simulink model "BTP_HEV_UDC_fInal_25_11_19"  (R2019a)
settings: Solver=VariableStepAuto  StartTime=0.0  StopTime=100  RelTol=1e-3
undefined symbols (not defined in the file): f_co, f_co2, f_hc, f_nox, f_tbrake_n_bpt, f_tbrake_t_bpt
libraries: fl_lib x100, nesl_utility x32, ee_lib x26, sdl_lib x17, simulink x5
(part 2 of 2)

== system BTP_HEV_UDC_fInal_25_11_19/Motor/Battery Subsystem/Battery Pack Subsystem/battery unit1 ==
  Capacitor : fl_lib/Electrical/Electrical Elements/Capacitor  c=5000 F  r=1e-6 Ohm  g=0 1/Ohm  i_specify=off  i_priority=None  i=0 A  i_nominal_specify=off  i_nominal_unit=A  i_nominal_value=1  v_specify=off  v_priority=None  v=0 V  v_nominal_specify=off  v_nominal_unit=V  v_nominal_value=1  vc_specify=off  vc_priority=High  vc=0 V  vc_nominal_specify=off  vc_nominal_unit=V  vc_nominal_value=1
  DC Voltage Source : ee_lib/Additional Components/SPICE Sources/DC Voltage Source  DC=4 V
      settings: SourceProductName=Simscape Electrical
  Resistor : fl_lib/Electrical/Electrical Elements/Resistor  R=.01 Ohm  i_specify=off  i_priority=None  i=0 A  i_nominal_specify=off  i_nominal_unit=A  i_nominal_value=1  v_specify=off  v_priority=None  v=0 V  v_nominal_specify=off  v_nominal_unit=V  v_nominal_value=1
  Resistor1 : fl_lib/Electrical/Electrical Elements/Resistor  R=.005 Ohm  i_specify=off  i_priority=None  i=0 A  i_nominal_specify=off  i_nominal_unit=A  i_nominal_value=1  v_specify=off  v_priority=None  v=0 V  v_nominal_specify=off  v_nominal_unit=V  v_nominal_value=1
  + : PMIOPort  Side=Right
  - : PMIOPort  Port=2  Side=Left
  connections:
  Resistor/LConn1 -- DC Voltage Source/LConn1
  -/RConn1 -- DC Voltage Source/RConn1
  +/RConn1 -- Capacitor/RConn1 -- Resistor1/RConn1
  Resistor1/LConn1 -- Capacitor/LConn1 -- Resistor/RConn1

== system BTP_HEV_UDC_fInal_25_11_19/Motor/Battery Subsystem/Battery Pack Subsystem/battery unit10 ==
  Capacitor : fl_lib/Electrical/Electrical Elements/Capacitor  c=5000 F  r=1e-6 Ohm  g=0 1/Ohm  i_specify=off  i_priority=None  i=0 A  i_nominal_specify=off  i_nominal_unit=A  i_nominal_value=1  v_specify=off  v_priority=None  v=0 V  v_nominal_specify=off  v_nominal_unit=V  v_nominal_value=1  vc_specify=off  vc_priority=High  vc=0 V  vc_nominal_specify=off  vc_nominal_unit=V  vc_nominal_value=1
  DC Voltage Source : ee_lib/Additional Components/SPICE Sources/DC Voltage Source  DC=4 V
      settings: SourceProductName=Simscape Electrical
  Resistor : fl_lib/Electrical/Electrical Elements/Resistor  R=.01 Ohm  i_specify=off  i_priority=None  i=0 A  i_nominal_specify=off  i_nominal_unit=A  i_nominal_value=1  v_specify=off  v_priority=None  v=0 V  v_nominal_specify=off  v_nominal_unit=V  v_nominal_value=1
  Resistor1 : fl_lib/Electrical/Electrical Elements/Resistor  R=.005 Ohm  i_specify=off  i_priority=None  i=0 A  i_nominal_specify=off  i_nominal_unit=A  i_nominal_value=1  v_specify=off  v_priority=None  v=0 V  v_nominal_specify=off  v_nominal_unit=V  v_nominal_value=1
  + : PMIOPort  Side=Right
  - : PMIOPort  Port=2  Side=Left
  connections:
  Resistor/RConn1 -- Capacitor/LConn1 -- Resistor1/LConn1
  Resistor1/RConn1 -- Capacitor/RConn1 -- +/RConn1
  -/RConn1 -- DC Voltage Source/RConn1
  Resistor/LConn1 -- DC Voltage Source/LConn1

== system BTP_HEV_UDC_fInal_25_11_19/Motor/Battery Subsystem/Battery Pack Subsystem/battery unit11 ==
  Capacitor : fl_lib/Electrical/Electrical Elements/Capacitor  c=5000 F  r=1e-6 Ohm  g=0 1/Ohm  i_specify=off  i_priority=None  i=0 A  i_nominal_specify=off  i_nominal_unit=A  i_nominal_value=1  v_specify=off  v_priority=None  v=0 V  v_nominal_specify=off  v_nominal_unit=V  v_nominal_value=1  vc_specify=off  vc_priority=High  vc=0 V  vc_nominal_specify=off  vc_nominal_unit=V  vc_nominal_value=1
  DC Voltage Source : ee_lib/Additional Components/SPICE Sources/DC Voltage Source  DC=4 V
      settings: SourceProductName=Simscape Electrical
  Resistor : fl_lib/Electrical/Electrical Elements/Resistor  R=.01 Ohm  i_specify=off  i_priority=None  i=0 A  i_nominal_specify=off  i_nominal_unit=A  i_nominal_value=1  v_specify=off  v_priority=None  v=0 V  v_nominal_specify=off  v_nominal_unit=V  v_nominal_value=1
  Resistor1 : fl_lib/Electrical/Electrical Elements/Resistor  R=.005 Ohm  i_specify=off  i_priority=None  i=0 A  i_nominal_specify=off  i_nominal_unit=A  i_nominal_value=1  v_specify=off  v_priority=None  v=0 V  v_nominal_specify=off  v_nominal_unit=V  v_nominal_value=1
  + : PMIOPort  Side=Right
  - : PMIOPort  Port=2  Side=Left
  connections:
  Resistor/LConn1 -- DC Voltage Source/LConn1
  -/RConn1 -- DC Voltage Source/RConn1
  +/RConn1 -- Capacitor/RConn1 -- Resistor1/RConn1
  Resistor1/LConn1 -- Capacitor/LConn1 -- Resistor/RConn1

== system BTP_HEV_UDC_fInal_25_11_19/Motor/Battery Subsystem/Battery Pack Subsystem/battery unit12 ==
  Capacitor : fl_lib/Electrical/Electrical Elements/Capacitor  c=5000 F  r=1e-6 Ohm  g=0 1/Ohm  i_specify=off  i_priority=None  i=0 A  i_nominal_specify=off  i_nominal_unit=A  i_nominal_value=1  v_specify=off  v_priority=None  v=0 V  v_nominal_specify=off  v_nominal_unit=V  v_nominal_value=1  vc_specify=off  vc_priority=High  vc=0 V  vc_nominal_specify=off  vc_nominal_unit=V  vc_nominal_value=1
  DC Voltage Source : ee_lib/Additional Components/SPICE Sources/DC Voltage Source  DC=4 V
      settings: SourceProductName=Simscape Electrical
  Resistor : fl_lib/Electrical/Electrical Elements/Resistor  R=.01 Ohm  i_specify=off  i_priority=None  i=0 A  i_nominal_specify=off  i_nominal_unit=A  i_nominal_value=1  v_specify=off  v_priority=None  v=0 V  v_nominal_specify=off  v_nominal_unit=V  v_nominal_value=1
  Resistor1 : fl_lib/Electrical/Electrical Elements/Resistor  R=.005 Ohm  i_specify=off  i_priority=None  i=0 A  i_nominal_specify=off  i_nominal_unit=A  i_nominal_value=1  v_specify=off  v_priority=None  v=0 V  v_nominal_specify=off  v_nominal_unit=V  v_nominal_value=1
  + : PMIOPort  Side=Right
  - : PMIOPort  Port=2  Side=Left
  connections:
  Resistor/RConn1 -- Capacitor/LConn1 -- Resistor1/LConn1
  Resistor1/RConn1 -- Capacitor/RConn1 -- +/RConn1
  -/RConn1 -- DC Voltage Source/RConn1
  Resistor/LConn1 -- DC Voltage Source/LConn1

== system BTP_HEV_UDC_fInal_25_11_19/Motor/Battery Subsystem/Battery Pack Subsystem/battery unit13 ==
  Capacitor : fl_lib/Electrical/Electrical Elements/Capacitor  c=5000 F  r=1e-6 Ohm  g=0 1/Ohm  i_specify=off  i_priority=None  i=0 A  i_nominal_specify=off  i_nominal_unit=A  i_nominal_value=1  v_specify=off  v_priority=None  v=0 V  v_nominal_specify=off  v_nominal_unit=V  v_nominal_value=1  vc_specify=off  vc_priority=High  vc=0 V  vc_nominal_specify=off  vc_nominal_unit=V  vc_nominal_value=1
  DC Voltage Source : ee_lib/Additional Components/SPICE Sources/DC Voltage Source  DC=.01 V
      settings: SourceProductName=Simscape Electrical
  Resistor : fl_lib/Electrical/Electrical Elements/Resistor  R=.01 Ohm  i_specify=off  i_priority=None  i=0 A  i_nominal_specify=off  i_nominal_unit=A  i_nominal_value=1  v_specify=off  v_priority=None  v=0 V  v_nominal_specify=off  v_nominal_unit=V  v_nominal_value=1
  Resistor1 : fl_lib/Electrical/Electrical Elements/Resistor  R=.005 Ohm  i_specify=off  i_priority=None  i=0 A  i_nominal_specify=off  i_nominal_unit=A  i_nominal_value=1  v_specify=off  v_priority=None  v=0 V  v_nominal_specify=off  v_nominal_unit=V  v_nominal_value=1
  + : PMIOPort  Side=Right
  - : PMIOPort  Port=2  Side=Left
  connections:
  Resistor/LConn1 -- DC Voltage Source/LConn1
  -/RConn1 -- DC Voltage Source/RConn1
  +/RConn1 -- Capacitor/RConn1 -- Resistor1/RConn1
  Resistor1/LConn1 -- Capacitor/LConn1 -- Resistor/RConn1

== system BTP_HEV_UDC_fInal_25_11_19/Motor/Battery Subsystem/Battery Pack Subsystem/battery unit14 ==
  Capacitor : fl_lib/Electrical/Electrical Elements/Capacitor  c=5000 F  r=1e-6 Ohm  g=0 1/Ohm  i_specify=off  i_priority=None  i=0 A  i_nominal_specify=off  i_nominal_unit=A  i_nominal_value=1  v_specify=off  v_priority=None  v=0 V  v_nominal_specify=off  v_nominal_unit=V  v_nominal_value=1  vc_specify=off  vc_priority=High  vc=0 V  vc_nominal_specify=off  vc_nominal_unit=V  vc_nominal_value=1
  DC Voltage Source : ee_lib/Additional Components/SPICE Sources/DC Voltage Source  DC=4 V
      settings: SourceProductName=Simscape Electrical
  Resistor : fl_lib/Electrical/Electrical Elements/Resistor  R=.01 Ohm  i_specify=off  i_priority=None  i=0 A  i_nominal_specify=off  i_nominal_unit=A  i_nominal_value=1  v_specify=off  v_priority=None  v=0 V  v_nominal_specify=off  v_nominal_unit=V  v_nominal_value=1
  Resistor1 : fl_lib/Electrical/Electrical Elements/Resistor  R=.005 Ohm  i_specify=off  i_priority=None  i=0 A  i_nominal_specify=off  i_nominal_unit=A  i_nominal_value=1  v_specify=off  v_priority=None  v=0 V  v_nominal_specify=off  v_nominal_unit=V  v_nominal_value=1
  + : PMIOPort  Side=Right
  - : PMIOPort  Port=2  Side=Left
  connections:
  Resistor/RConn1 -- Capacitor/LConn1 -- Resistor1/LConn1
  Resistor1/RConn1 -- Capacitor/RConn1 -- +/RConn1
  -/RConn1 -- DC Voltage Source/RConn1
  Resistor/LConn1 -- DC Voltage Source/LConn1

== system BTP_HEV_UDC_fInal_25_11_19/Motor/Battery Subsystem/Battery Pack Subsystem/battery unit15 ==
  Capacitor : fl_lib/Electrical/Electrical Elements/Capacitor  c=5000 F  r=1e-6 Ohm  g=0 1/Ohm  i_specify=off  i_priority=None  i=0 A  i_nominal_specify=off  i_nominal_unit=A  i_nominal_value=1  v_specify=off  v_priority=None  v=0 V  v_nominal_specify=off  v_nominal_unit=V  v_nominal_value=1  vc_specify=off  vc_priority=High  vc=0 V  vc_nominal_specify=off  vc_nominal_unit=V  vc_nominal_value=1
  DC Voltage Source : ee_lib/Additional Components/SPICE Sources/DC Voltage Source  DC=4 V
      settings: SourceProductName=Simscape Electrical
  Resistor : fl_lib/Electrical/Electrical Elements/Resistor  R=.01 Ohm  i_specify=off  i_priority=None  i=0 A  i_nominal_specify=off  i_nominal_unit=A  i_nominal_value=1  v_specify=off  v_priority=None  v=0 V  v_nominal_specify=off  v_nominal_unit=V  v_nominal_value=1
  Resistor1 : fl_lib/Electrical/Electrical Elements/Resistor  R=.005 Ohm  i_specify=off  i_priority=None  i=0 A  i_nominal_specify=off  i_nominal_unit=A  i_nominal_value=1  v_specify=off  v_priority=None  v=0 V  v_nominal_specify=off  v_nominal_unit=V  v_nominal_value=1
  + : PMIOPort  Side=Right
  - : PMIOPort  Port=2  Side=Left
  connections:
  Resistor/LConn1 -- DC Voltage Source/LConn1
  -/RConn1 -- DC Voltage Source/RConn1
  +/RConn1 -- Capacitor/RConn1 -- Resistor1/RConn1
  Resistor1/LConn1 -- Capacitor/LConn1 -- Resistor/RConn1

== system BTP_HEV_UDC_fInal_25_11_19/Motor/Battery Subsystem/Battery Pack Subsystem/battery unit16 ==
  Capacitor : fl_lib/Electrical/Electrical Elements/Capacitor  c=5000 F  r=1e-6 Ohm  g=0 1/Ohm  i_specify=off  i_priority=None  i=0 A  i_nominal_specify=off  i_nominal_unit=A  i_nominal_value=1  v_specify=off  v_priority=None  v=0 V  v_nominal_specify=off  v_nominal_unit=V  v_nominal_value=1  vc_specify=off  vc_priority=High  vc=0 V  vc_nominal_specify=off  vc_nominal_unit=V  vc_nominal_value=1
  DC Voltage Source : ee_lib/Additional Components/SPICE Sources/DC Voltage Source  DC=4 V
      settings: SourceProductName=Simscape Electrical
  Resistor : fl_lib/Electrical/Electrical Elements/Resistor  R=.01 Ohm  i_specify=off  i_priority=None  i=0 A  i_nominal_specify=off  i_nominal_unit=A  i_nominal_value=1  v_specify=off  v_priority=None  v=0 V  v_nominal_specify=off  v_nominal_unit=V  v_nominal_value=1
  Resistor1 : fl_lib/Electrical/Electrical Elements/Resistor  R=.005 Ohm  i_specify=off  i_priority=None  i=0 A  i_nominal_specify=off  i_nominal_unit=A  i_nominal_value=1  v_specify=off  v_priority=None  v=0 V  v_nominal_specify=off  v_nominal_unit=V  v_nominal_value=1
  + : PMIOPort  Side=Right
  - : PMIOPort  Port=2  Side=Left
  connections:
  Resistor/RConn1 -- Capacitor/LConn1 -- Resistor1/LConn1
  Resistor1/RConn1 -- Capacitor/RConn1 -- +/RConn1
  -/RConn1 -- DC Voltage Source/RConn1
  Resistor/LConn1 -- DC Voltage Source/LConn1

== system BTP_HEV_UDC_fInal_25_11_19/Motor/Battery Subsystem/Battery Pack Subsystem/battery unit17 ==
  Capacitor : fl_lib/Electrical/Electrical Elements/Capacitor  c=5000 F  r=1e-6 Ohm  g=0 1/Ohm  i_specify=off  i_priority=None  i=0 A  i_nominal_specify=off  i_nominal_unit=A  i_nominal_value=1  v_specify=off  v_priority=None  v=0 V  v_nominal_specify=off  v_nominal_unit=V  v_nominal_value=1  vc_specify=off  vc_priority=High  vc=0 V  vc_nominal_specify=off  vc_nominal_unit=V  vc_nominal_value=1
  DC Voltage Source : ee_lib/Additional Components/SPICE Sources/DC Voltage Source  DC=4 V
      settings: SourceProductName=Simscape Electrical
  Resistor : fl_lib/Electrical/Electrical Elements/Resistor  R=.01 Ohm  i_specify=off  i_priority=None  i=0 A  i_nominal_specify=off  i_nominal_unit=A  i_nominal_value=1  v_specify=off  v_priority=None  v=0 V  v_nominal_specify=off  v_nominal_unit=V  v_nominal_value=1
  Resistor1 : fl_lib/Electrical/Electrical Elements/Resistor  R=.005 Ohm  i_specify=off  i_priority=None  i=0 A  i_nominal_specify=off  i_nominal_unit=A  i_nominal_value=1  v_specify=off  v_priority=None  v=0 V  v_nominal_specify=off  v_nominal_unit=V  v_nominal_value=1
  + : PMIOPort  Side=Right
  - : PMIOPort  Port=2  Side=Left
  connections:
  Resistor/LConn1 -- DC Voltage Source/LConn1
  -/RConn1 -- DC Voltage Source/RConn1
  +/RConn1 -- Capacitor/RConn1 -- Resistor1/RConn1
  Resistor1/LConn1 -- Capacitor/LConn1 -- Resistor/RConn1

== system BTP_HEV_UDC_fInal_25_11_19/Motor/Battery Subsystem/Battery Pack Subsystem/battery unit18 ==
  Capacitor : fl_lib/Electrical/Electrical Elements/Capacitor  c=5000 F  r=1e-6 Ohm  g=0 1/Ohm  i_specify=off  i_priority=None  i=0 A  i_nominal_specify=off  i_nominal_unit=A  i_nominal_value=1  v_specify=off  v_priority=None  v=0 V  v_nominal_specify=off  v_nominal_unit=V  v_nominal_value=1  vc_specify=off  vc_priority=High  vc=0 V  vc_nominal_specify=off  vc_nominal_unit=V  vc_nominal_value=1
  DC Voltage Source : ee_lib/Additional Components/SPICE Sources/DC Voltage Source  DC=4 V
      settings: SourceProductName=Simscape Electrical
  Resistor : fl_lib/Electrical/Electrical Elements/Resistor  R=.01 Ohm  i_specify=off  i_priority=None  i=0 A  i_nominal_specify=off  i_nominal_unit=A  i_nominal_value=1  v_specify=off  v_priority=None  v=0 V  v_nominal_specify=off  v_nominal_unit=V  v_nominal_value=1
  Resistor1 : fl_lib/Electrical/Electrical Elements/Resistor  R=.005 Ohm  i_specify=off  i_priority=None  i=0 A  i_nominal_specify=off  i_nominal_unit=A  i_nominal_value=1  v_specify=off  v_priority=None  v=0 V  v_nominal_specify=off  v_nominal_unit=V  v_nominal_value=1
  + : PMIOPort  Side=Right
  - : PMIOPort  Port=2  Side=Left
  connections:
  Resistor/RConn1 -- Capacitor/LConn1 -- Resistor1/LConn1
  Resistor1/RConn1 -- Capacitor/RConn1 -- +/RConn1
  -/RConn1 -- DC Voltage Source/RConn1
  Resistor/LConn1 -- DC Voltage Source/LConn1

== system BTP_HEV_UDC_fInal_25_11_19/Motor/Battery Subsystem/Battery Pack Subsystem/battery unit19 ==
  Capacitor : fl_lib/Electrical/Electrical Elements/Capacitor  c=5000 F  r=1e-6 Ohm  g=0 1/Ohm  i_specify=off  i_priority=None  i=0 A  i_nominal_specify=off  i_nominal_unit=A  i_nominal_value=1  v_specify=off  v_priority=None  v=0 V  v_nominal_specify=off  v_nominal_unit=V  v_nominal_value=1  vc_specify=off  vc_priority=High  vc=0 V  vc_nominal_specify=off  vc_nominal_unit=V  vc_nominal_value=1
  DC Voltage Source : ee_lib/Additional Components/SPICE Sources/DC Voltage Source  DC=4 V
      settings: SourceProductName=Simscape Electrical
  Resistor : fl_lib/Electrical/Electrical Elements/Resistor  R=.01 Ohm  i_specify=off  i_priority=None  i=0 A  i_nominal_specify=off  i_nominal_unit=A  i_nominal_value=1  v_specify=off  v_priority=None  v=0 V  v_nominal_specify=off  v_nominal_unit=V  v_nominal_value=1
  Resistor1 : fl_lib/Electrical/Electrical Elements/Resistor  R=.005 Ohm  i_specify=off  i_priority=None  i=0 A  i_nominal_specify=off  i_nominal_unit=A  i_nominal_value=1  v_specify=off  v_priority=None  v=0 V  v_nominal_specify=off  v_nominal_unit=V  v_nominal_value=1
  + : PMIOPort  Side=Right
  - : PMIOPort  Port=2  Side=Left
  connections:
  Resistor/LConn1 -- DC Voltage Source/LConn1
  -/RConn1 -- DC Voltage Source/RConn1
  +/RConn1 -- Capacitor/RConn1 -- Resistor1/RConn1
  Resistor1/LConn1 -- Capacitor/LConn1 -- Resistor/RConn1

== system BTP_HEV_UDC_fInal_25_11_19/Motor/Battery Subsystem/Battery Pack Subsystem/battery unit2 ==
  Capacitor : fl_lib/Electrical/Electrical Elements/Capacitor  c=5000 F  r=1e-6 Ohm  g=0 1/Ohm  i_specify=off  i_priority=None  i=0 A  i_nominal_specify=off  i_nominal_unit=A  i_nominal_value=1  v_specify=off  v_priority=None  v=0 V  v_nominal_specify=off  v_nominal_unit=V  v_nominal_value=1  vc_specify=off  vc_priority=High  vc=0 V  vc_nominal_specify=off  vc_nominal_unit=V  vc_nominal_value=1
  DC Voltage Source : ee_lib/Additional Components/SPICE Sources/DC Voltage Source  DC=4 V
      settings: SourceProductName=Simscape Electrical
  Resistor : fl_lib/Electrical/Electrical Elements/Resistor  R=.01 Ohm  i_specify=off  i_priority=None  i=0 A  i_nominal_specify=off  i_nominal_unit=A  i_nominal_value=1  v_specify=off  v_priority=None  v=0 V  v_nominal_specify=off  v_nominal_unit=V  v_nominal_value=1
  Resistor1 : fl_lib/Electrical/Electrical Elements/Resistor  R=.005 Ohm  i_specify=off  i_priority=None  i=0 A  i_nominal_specify=off  i_nominal_unit=A  i_nominal_value=1  v_specify=off  v_priority=None  v=0 V  v_nominal_specify=off  v_nominal_unit=V  v_nominal_value=1
  + : PMIOPort  Side=Right
  - : PMIOPort  Port=2  Side=Left
  connections:
  Resistor/RConn1 -- Capacitor/LConn1 -- Resistor1/LConn1
  Resistor1/RConn1 -- Capacitor/RConn1 -- +/RConn1
  -/RConn1 -- DC Voltage Source/RConn1
  Resistor/LConn1 -- DC Voltage Source/LConn1

== system BTP_HEV_UDC_fInal_25_11_19/Motor/Battery Subsystem/Battery Pack Subsystem/battery unit20 ==
  Capacitor : fl_lib/Electrical/Electrical Elements/Capacitor  c=5000 F  r=1e-6 Ohm  g=0 1/Ohm  i_specify=off  i_priority=None  i=0 A  i_nominal_specify=off  i_nominal_unit=A  i_nominal_value=1  v_specify=off  v_priority=None  v=0 V  v_nominal_specify=off  v_nominal_unit=V  v_nominal_value=1  vc_specify=off  vc_priority=High  vc=0 V  vc_nominal_specify=off  vc_nominal_unit=V  vc_nominal_value=1
  DC Voltage Source : ee_lib/Additional Components/SPICE Sources/DC Voltage Source  DC=4 V
      settings: SourceProductName=Simscape Electrical
  Resistor : fl_lib/Electrical/Electrical Elements/Resistor  R=.01 Ohm  i_specify=off  i_priority=None  i=0 A  i_nominal_specify=off  i_nominal_unit=A  i_nominal_value=1  v_specify=off  v_priority=None  v=0 V  v_nominal_specify=off  v_nominal_unit=V  v_nominal_value=1
  Resistor1 : fl_lib/Electrical/Electrical Elements/Resistor  R=.005 Ohm  i_specify=off  i_priority=None  i=0 A  i_nominal_specify=off  i_nominal_unit=A  i_nominal_value=1  v_specify=off  v_priority=None  v=0 V  v_nominal_specify=off  v_nominal_unit=V  v_nominal_value=1
  + : PMIOPort  Side=Right
  - : PMIOPort  Port=2  Side=Left
  connections:
  Resistor/RConn1 -- Capacitor/LConn1 -- Resistor1/LConn1
  Resistor1/RConn1 -- Capacitor/RConn1 -- +/RConn1
  -/RConn1 -- DC Voltage Source/RConn1
  Resistor/LConn1 -- DC Voltage Source/LConn1

== system BTP_HEV_UDC_fInal_25_11_19/Motor/Battery Subsystem/Battery Pack Subsystem/battery unit21 ==
  Capacitor : fl_lib/Electrical/Electrical Elements/Capacitor  c=5000 F  r=1e-6 Ohm  g=0 1/Ohm  i_specify=off  i_priority=None  i=0 A  i_nominal_specify=off  i_nominal_unit=A  i_nominal_value=1  v_specify=off  v_priority=None  v=0 V  v_nominal_specify=off  v_nominal_unit=V  v_nominal_value=1  vc_specify=off  vc_priority=High  vc=0 V  vc_nominal_specify=off  vc_nominal_unit=V  vc_nominal_value=1
  DC Voltage Source : ee_lib/Additional Components/SPICE Sources/DC Voltage Source  DC=4 V
      settings: SourceProductName=Simscape Electrical
  Resistor : fl_lib/Electrical/Electrical Elements/Resistor  R=.01 Ohm  i_specify=off  i_priority=None  i=0 A  i_nominal_specify=off  i_nominal_unit=A  i_nominal_value=1  v_specify=off  v_priority=None  v=0 V  v_nominal_specify=off  v_nominal_unit=V  v_nominal_value=1
  Resistor1 : fl_lib/Electrical/Electrical Elements/Resistor  R=.005 Ohm  i_specify=off  i_priority=None  i=0 A  i_nominal_specify=off  i_nominal_unit=A  i_nominal_value=1  v_specify=off  v_priority=None  v=0 V  v_nominal_specify=off  v_nominal_unit=V  v_nominal_value=1
  + : PMIOPort  Side=Right
  - : PMIOPort  Port=2  Side=Left
  connections:
  Resistor/LConn1 -- DC Voltage Source/LConn1
  -/RConn1 -- DC Voltage Source/RConn1
  +/RConn1 -- Capacitor/RConn1 -- Resistor1/RConn1
  Resistor1/LConn1 -- Capacitor/LConn1 -- Resistor/RConn1

== system BTP_HEV_UDC_fInal_25_11_19/Motor/Battery Subsystem/Battery Pack Subsystem/battery unit22 ==
  Capacitor : fl_lib/Electrical/Electrical Elements/Capacitor  c=5000 F  r=1e-6 Ohm  g=0 1/Ohm  i_specify=off  i_priority=None  i=0 A  i_nominal_specify=off  i_nominal_unit=A  i_nominal_value=1  v_specify=off  v_priority=None  v=0 V  v_nominal_specify=off  v_nominal_unit=V  v_nominal_value=1  vc_specify=off  vc_priority=High  vc=0 V  vc_nominal_specify=off  vc_nominal_unit=V  vc_nominal_value=1
  DC Voltage Source : ee_lib/Additional Components/SPICE Sources/DC Voltage Source  DC=4 V
      settings: SourceProductName=Simscape Electrical
  Resistor : fl_lib/Electrical/Electrical Elements/Resistor  R=.01 Ohm  i_specify=off  i_priority=None  i=0 A  i_nominal_specify=off  i_nominal_unit=A  i_nominal_value=1  v_specify=off  v_priority=None  v=0 V  v_nominal_specify=off  v_nominal_unit=V  v_nominal_value=1
  Resistor1 : fl_lib/Electrical/Electrical Elements/Resistor  R=.005 Ohm  i_specify=off  i_priority=None  i=0 A  i_nominal_specify=off  i_nominal_unit=A  i_nominal_value=1  v_specify=off  v_priority=None  v=0 V  v_nominal_specify=off  v_nominal_unit=V  v_nominal_value=1
  + : PMIOPort  Side=Right
  - : PMIOPort  Port=2  Side=Left
  connections:
  Resistor/RConn1 -- Capacitor/LConn1 -- Resistor1/LConn1
  Resistor1/RConn1 -- Capacitor/RConn1 -- +/RConn1
  -/RConn1 -- DC Voltage Source/RConn1
  Resistor/LConn1 -- DC Voltage Source/LConn1

== system BTP_HEV_UDC_fInal_25_11_19/Motor/Battery Subsystem/Battery Pack Subsystem/battery unit23 ==
  Capacitor : fl_lib/Electrical/Electrical Elements/Capacitor  c=5000 F  r=1e-6 Ohm  g=0 1/Ohm  i_specify=off  i_priority=None  i=0 A  i_nominal_specify=off  i_nominal_unit=A  i_nominal_value=1  v_specify=off  v_priority=None  v=0 V  v_nominal_specify=off  v_nominal_unit=V  v_nominal_value=1  vc_specify=off  vc_priority=High  vc=0 V  vc_nominal_specify=off  vc_nominal_unit=V  vc_nominal_value=1
  DC Voltage Source : ee_lib/Additional Components/SPICE Sources/DC Voltage Source  DC=4 V
      settings: SourceProductName=Simscape Electrical
  Resistor : fl_lib/Electrical/Electrical Elements/Resistor  R=.01 Ohm  i_specify=off  i_priority=None  i=0 A  i_nominal_specify=off  i_nominal_unit=A  i_nominal_value=1  v_specify=off  v_priority=None  v=0 V  v_nominal_specify=off  v_nominal_unit=V  v_nominal_value=1
  Resistor1 : fl_lib/Electrical/Electrical Elements/Resistor  R=.005 Ohm  i_specify=off  i_priority=None  i=0 A  i_nominal_specify=off  i_nominal_unit=A  i_nominal_value=1  v_specify=off  v_priority=None  v=0 V  v_nominal_specify=off  v_nominal_unit=V  v_nominal_value=1
  + : PMIOPort  Side=Right
  - : PMIOPort  Port=2  Side=Left
  connections:
  Resistor/LConn1 -- DC Voltage Source/LConn1
  -/RConn1 -- DC Voltage Source/RConn1
  +/RConn1 -- Capacitor/RConn1 -- Resistor1/RConn1
  Resistor1/LConn1 -- Capacitor/LConn1 -- Resistor/RConn1

== system BTP_HEV_UDC_fInal_25_11_19/Motor/Battery Subsystem/Battery Pack Subsystem/battery unit24 ==
  Capacitor : fl_lib/Electrical/Electrical Elements/Capacitor  c=5000 F  r=1e-6 Ohm  g=0 1/Ohm  i_specify=off  i_priority=None  i=0 A  i_nominal_specify=off  i_nominal_unit=A  i_nominal_value=1  v_specify=off  v_priority=None  v=0 V  v_nominal_specify=off  v_nominal_unit=V  v_nominal_value=1  vc_specify=off  vc_priority=High  vc=0 V  vc_nominal_specify=off  vc_nominal_unit=V  vc_nominal_value=1
  DC Voltage Source : ee_lib/Additional Components/SPICE Sources/DC Voltage Source  DC=4 V
      settings: SourceProductName=Simscape Electrical
  Resistor : fl_lib/Electrical/Electrical Elements/Resistor  R=.01 Ohm  i_specify=off  i_priority=None  i=0 A  i_nominal_specify=off  i_nominal_unit=A  i_nominal_value=1  v_specify=off  v_priority=None  v=0 V  v_nominal_specify=off  v_nominal_unit=V  v_nominal_value=1
  Resistor1 : fl_lib/Electrical/Electrical Elements/Resistor  R=.005 Ohm  i_specify=off  i_priority=None  i=0 A  i_nominal_specify=off  i_nominal_unit=A  i_nominal_value=1  v_specify=off  v_priority=None  v=0 V  v_nominal_specify=off  v_nominal_unit=V  v_nominal_value=1
  + : PMIOPort  Side=Right
  - : PMIOPort  Port=2  Side=Left
  connections:
  Resistor/RConn1 -- Capacitor/LConn1 -- Resistor1/LConn1
  Resistor1/RConn1 -- Capacitor/RConn1 -- +/RConn1
  -/RConn1 -- DC Voltage Source/RConn1
  Resistor/LConn1 -- DC Voltage Source/LConn1

== system BTP_HEV_UDC_fInal_25_11_19/Motor/Battery Subsystem/Battery Pack Subsystem/battery unit3 ==
  Capacitor : fl_lib/Electrical/Electrical Elements/Capacitor  c=5000 F  r=1e-6 Ohm  g=0 1/Ohm  i_specify=off  i_priority=None  i=0 A  i_nominal_specify=off  i_nominal_unit=A  i_nominal_value=1  v_specify=off  v_priority=None  v=0 V  v_nominal_specify=off  v_nominal_unit=V  v_nominal_value=1  vc_specify=off  vc_priority=High  vc=0 V  vc_nominal_specify=off  vc_nominal_unit=V  vc_nominal_value=1
  DC Voltage Source : ee_lib/Additional Components/SPICE Sources/DC Voltage Source  DC=4 V
      settings: SourceProductName=Simscape Electrical
  Resistor : fl_lib/Electrical/Electrical Elements/Resistor  R=.01 Ohm  i_specify=off  i_priority=None  i=0 A  i_nominal_specify=off  i_nominal_unit=A  i_nominal_value=1  v_specify=off  v_priority=None  v=0 V  v_nominal_specify=off  v_nominal_unit=V  v_nominal_value=1
  Resistor1 : fl_lib/Electrical/Electrical Elements/Resistor  R=.005 Ohm  i_specify=off  i_priority=None  i=0 A  i_nominal_specify=off  i_nominal_unit=A  i_nominal_value=1  v_specify=off  v_priority=None  v=0 V  v_nominal_specify=off  v_nominal_unit=V  v_nominal_value=1
  + : PMIOPort  Side=Right
  - : PMIOPort  Port=2  Side=Left
  connections:
  Resistor/LConn1 -- DC Voltage Source/LConn1
  -/RConn1 -- DC Voltage Source/RConn1
  +/RConn1 -- Capacitor/RConn1 -- Resistor1/RConn1
  Resistor1/LConn1 -- Capacitor/LConn1 -- Resistor/RConn1

== system BTP_HEV_UDC_fInal_25_11_19/Motor/Battery Subsystem/Battery Pack Subsystem/battery unit4 ==
  Capacitor : fl_lib/Electrical/Electrical Elements/Capacitor  c=5000 F  r=1e-6 Ohm  g=0 1/Ohm  i_specify=off  i_priority=None  i=0 A  i_nominal_specify=off  i_nominal_unit=A  i_nominal_value=1  v_specify=off  v_priority=None  v=0 V  v_nominal_specify=off  v_nominal_unit=V  v_nominal_value=1  vc_specify=off  vc_priority=High  vc=0 V  vc_nominal_specify=off  vc_nominal_unit=V  vc_nominal_value=1
  DC Voltage Source : ee_lib/Additional Components/SPICE Sources/DC Voltage Source  DC=4 V
      settings: SourceProductName=Simscape Electrical
  Resistor : fl_lib/Electrical/Electrical Elements/Resistor  R=.01 Ohm  i_specify=off  i_priority=None  i=0 A  i_nominal_specify=off  i_nominal_unit=A  i_nominal_value=1  v_specify=off  v_priority=None  v=0 V  v_nominal_specify=off  v_nominal_unit=V  v_nominal_value=1
  Resistor1 : fl_lib/Electrical/Electrical Elements/Resistor  R=.005 Ohm  i_specify=off  i_priority=None  i=0 A  i_nominal_specify=off  i_nominal_unit=A  i_nominal_value=1  v_specify=off  v_priority=None  v=0 V  v_nominal_specify=off  v_nominal_unit=V  v_nominal_value=1
  + : PMIOPort  Side=Right
  - : PMIOPort  Port=2  Side=Left
  connections:
  Resistor/RConn1 -- Capacitor/LConn1 -- Resistor1/LConn1
  Resistor1/RConn1 -- Capacitor/RConn1 -- +/RConn1
  -/RConn1 -- DC Voltage Source/RConn1
  Resistor/LConn1 -- DC Voltage Source/LConn1

== system BTP_HEV_UDC_fInal_25_11_19/Motor/Battery Subsystem/Battery Pack Subsystem/battery unit5 ==
  Capacitor : fl_lib/Electrical/Electrical Elements/Capacitor  c=5000 F  r=1e-6 Ohm  g=0 1/Ohm  i_specify=off  i_priority=None  i=0 A  i_nominal_specify=off  i_nominal_unit=A  i_nominal_value=1  v_specify=off  v_priority=None  v=0 V  v_nominal_specify=off  v_nominal_unit=V  v_nominal_value=1  vc_specify=off  vc_priority=High  vc=0 V  vc_nominal_specify=off  vc_nominal_unit=V  vc_nominal_value=1
  DC Voltage Source : ee_lib/Additional Components/SPICE Sources/DC Voltage Source  DC=4 V
      settings: SourceProductName=Simscape Electrical
  Resistor : fl_lib/Electrical/Electrical Elements/Resistor  R=.01 Ohm  i_specify=off  i_priority=None  i=0 A  i_nominal_specify=off  i_nominal_unit=A  i_nominal_value=1  v_specify=off  v_priority=None  v=0 V  v_nominal_specify=off  v_nominal_unit=V  v_nominal_value=1
  Resistor1 : fl_lib/Electrical/Electrical Elements/Resistor  R=.005 Ohm  i_specify=off  i_priority=None  i=0 A  i_nominal_specify=off  i_nominal_unit=A  i_nominal_value=1  v_specify=off  v_priority=None  v=0 V  v_nominal_specify=off  v_nominal_unit=V  v_nominal_value=1
  + : PMIOPort  Side=Right
  - : PMIOPort  Port=2  Side=Left
  connections:
  Resistor/LConn1 -- DC Voltage Source/LConn1
  -/RConn1 -- DC Voltage Source/RConn1
  +/RConn1 -- Capacitor/RConn1 -- Resistor1/RConn1
  Resistor1/LConn1 -- Capacitor/LConn1 -- Resistor/RConn1

== system BTP_HEV_UDC_fInal_25_11_19/Motor/Battery Subsystem/Battery Pack Subsystem/battery unit6 ==
  Capacitor : fl_lib/Electrical/Electrical Elements/Capacitor  c=5000 F  r=1e-6 Ohm  g=0 1/Ohm  i_specify=off  i_priority=None  i=0 A  i_nominal_specify=off  i_nominal_unit=A  i_nominal_value=1  v_specify=off  v_priority=None  v=0 V  v_nominal_specify=off  v_nominal_unit=V  v_nominal_value=1  vc_specify=off  vc_priority=High  vc=0 V  vc_nominal_specify=off  vc_nominal_unit=V  vc_nominal_value=1
  DC Voltage Source : ee_lib/Additional Components/SPICE Sources/DC Voltage Source  DC=4 V
      settings: SourceProductName=Simscape Electrical
  Resistor : fl_lib/Electrical/Electrical Elements/Resistor  R=.01 Ohm  i_specify=off  i_priority=None  i=0 A  i_nominal_specify=off  i_nominal_unit=A  i_nominal_value=1  v_specify=off  v_priority=None  v=0 V  v_nominal_specify=off  v_nominal_unit=V  v_nominal_value=1
  Resistor1 : fl_lib/Electrical/Electrical Elements/Resistor  R=.005 Ohm  i_specify=off  i_priority=None  i=0 A  i_nominal_specify=off  i_nominal_unit=A  i_nominal_value=1  v_specify=off  v_priority=None  v=0 V  v_nominal_specify=off  v_nominal_unit=V  v_nominal_value=1
  + : PMIOPort  Side=Right
  - : PMIOPort  Port=2  Side=Left
  connections:
  Resistor/RConn1 -- Capacitor/LConn1 -- Resistor1/LConn1
  Resistor1/RConn1 -- Capacitor/RConn1 -- +/RConn1
  -/RConn1 -- DC Voltage Source/RConn1
  Resistor/LConn1 -- DC Voltage Source/LConn1

== system BTP_HEV_UDC_fInal_25_11_19/Motor/Battery Subsystem/Battery Pack Subsystem/battery unit7 ==
  Capacitor : fl_lib/Electrical/Electrical Elements/Capacitor  c=5000 F  r=1e-6 Ohm  g=0 1/Ohm  i_specify=off  i_priority=None  i=0 A  i_nominal_specify=off  i_nominal_unit=A  i_nominal_value=1  v_specify=off  v_priority=None  v=0 V  v_nominal_specify=off  v_nominal_unit=V  v_nominal_value=1  vc_specify=off  vc_priority=High  vc=0 V  vc_nominal_specify=off  vc_nominal_unit=V  vc_nominal_value=1
  DC Voltage Source : ee_lib/Additional Components/SPICE Sources/DC Voltage Source  DC=4 V
      settings: SourceProductName=Simscape Electrical
  Resistor : fl_lib/Electrical/Electrical Elements/Resistor  R=.01 Ohm  i_specify=off  i_priority=None  i=0 A  i_nominal_specify=off  i_nominal_unit=A  i_nominal_value=1  v_specify=off  v_priority=None  v=0 V  v_nominal_specify=off  v_nominal_unit=V  v_nominal_value=1
  Resistor1 : fl_lib/Electrical/Electrical Elements/Resistor  R=.005 Ohm  i_specify=off  i_priority=None  i=0 A  i_nominal_specify=off  i_nominal_unit=A  i_nominal_value=1  v_specify=off  v_priority=None  v=0 V  v_nominal_specify=off  v_nominal_unit=V  v_nominal_value=1
  + : PMIOPort  Side=Right
  - : PMIOPort  Port=2  Side=Left
  connections:
  Resistor/LConn1 -- DC Voltage Source/LConn1
  -/RConn1 -- DC Voltage Source/RConn1
  +/RConn1 -- Capacitor/RConn1 -- Resistor1/RConn1
  Resistor1/LConn1 -- Capacitor/LConn1 -- Resistor/RConn1

== system BTP_HEV_UDC_fInal_25_11_19/Motor/Battery Subsystem/Battery Pack Subsystem/battery unit8 ==
  Capacitor : fl_lib/Electrical/Electrical Elements/Capacitor  c=5000 F  r=1e-6 Ohm  g=0 1/Ohm  i_specify=off  i_priority=None  i=0 A  i_nominal_specify=off  i_nominal_unit=A  i_nominal_value=1  v_specify=off  v_priority=None  v=0 V  v_nominal_specify=off  v_nominal_unit=V  v_nominal_value=1  vc_specify=off  vc_priority=High  vc=0 V  vc_nominal_specify=off  vc_nominal_unit=V  vc_nominal_value=1
  DC Voltage Source : ee_lib/Additional Components/SPICE Sources/DC Voltage Source  DC=4 V
      settings: SourceProductName=Simscape Electrical
  Resistor : fl_lib/Electrical/Electrical Elements/Resistor  R=0.01 Ohm  i_specify=off  i_priority=None  i=0 A  i_nominal_specify=off  i_nominal_unit=A  i_nominal_value=1  v_specify=off  v_priority=None  v=0 V  v_nominal_specify=off  v_nominal_unit=V  v_nominal_value=1
  Resistor1 : fl_lib/Electrical/Electrical Elements/Resistor  R=.005 Ohm  i_specify=off  i_priority=None  i=0 A  i_nominal_specify=off  i_nominal_unit=A  i_nominal_value=1  v_specify=off  v_priority=None  v=0 V  v_nominal_specify=off  v_nominal_unit=V  v_nominal_value=1
  + : PMIOPort  Side=Right
  - : PMIOPort  Port=2  Side=Left
  connections:
  Resistor/RConn1 -- Capacitor/LConn1 -- Resistor1/LConn1
  Resistor1/RConn1 -- Capacitor/RConn1 -- +/RConn1
  -/RConn1 -- DC Voltage Source/RConn1
  Resistor/LConn1 -- DC Voltage Source/LConn1

== system BTP_HEV_UDC_fInal_25_11_19/Motor/Battery Subsystem/Battery Pack Subsystem/battery unit9 ==
  Capacitor : fl_lib/Electrical/Electrical Elements/Capacitor  c=5000 F  r=1e-6 Ohm  g=0 1/Ohm  i_specify=off  i_priority=None  i=0 A  i_nominal_specify=off  i_nominal_unit=A  i_nominal_value=1  v_specify=off  v_priority=None  v=0 V  v_nominal_specify=off  v_nominal_unit=V  v_nominal_value=1  vc_specify=off  vc_priority=High  vc=0 V  vc_nominal_specify=off  vc_nominal_unit=V  vc_nominal_value=1
  DC Voltage Source : ee_lib/Additional Components/SPICE Sources/DC Voltage Source  DC=4 V
      settings: SourceProductName=Simscape Electrical
  Resistor : fl_lib/Electrical/Electrical Elements/Resistor  R=.01 Ohm  i_specify=off  i_priority=None  i=0 A  i_nominal_specify=off  i_nominal_unit=A  i_nominal_value=1  v_specify=off  v_priority=None  v=0 V  v_nominal_specify=off  v_nominal_unit=V  v_nominal_value=1
  Resistor1 : fl_lib/Electrical/Electrical Elements/Resistor  R=.005 Ohm  i_specify=off  i_priority=None  i=0 A  i_nominal_specify=off  i_nominal_unit=A  i_nominal_value=1  v_specify=off  v_priority=None  v=0 V  v_nominal_specify=off  v_nominal_unit=V  v_nominal_value=1
  + : PMIOPort  Side=Right
  - : PMIOPort  Port=2  Side=Left
  connections:
  Resistor/LConn1 -- DC Voltage Source/LConn1
  -/RConn1 -- DC Voltage Source/RConn1
  +/RConn1 -- Capacitor/RConn1 -- Resistor1/RConn1
  Resistor1/LConn1 -- Capacitor/LConn1 -- Resistor/RConn1

== stateflow chart BTP_HEV_UDC_fInal_25_11_19/Drive Control/Chart ==
  state Motion_Mode
    state Start_Mode
      entry: Engine_out=0;
      Motor_out=1;
    state Highway_mode
      entry: Engine_out=1;
      state High_demand
        entry: Motor_out=2;
      state Cruising_Mode
        entry: Motor_out=0;
      (default) -> Motion_Mode.Highway_mode.High_demand
      Motion_Mode.Highway_mode.High_demand -> Motion_Mode.Highway_mode.Cruising_Mode : [30<speed&&speed<120&&acc<1.5]
      Motion_Mode.Highway_mode.Cruising_Mode -> Motion_Mode.Highway_mode.High_demand : [30>=speed||speed>=120||acc>=1.5]
    state Normal_Mode
      entry: Engine_out=1;
      state High_demand
        entry: Motor_out=2;
      state Cruising_Mode
        entry: Motor_out=0;
      (default) -> Motion_Mode.Normal_Mode.High_demand
      Motion_Mode.Normal_Mode.Cruising_Mode -> Motion_Mode.Normal_Mode.High_demand : [speed>=120||acc>=2]
      Motion_Mode.Normal_Mode.High_demand -> Motion_Mode.Normal_Mode.Cruising_Mode : [speed<120&&acc<2]
    Motion_Mode.Start_Mode -> Highway_mode [order 2] : [UDC==0]
    Motion_Mode.Start_Mode -> Motion_Mode.Normal_Mode [order 1] : [speed>=30&&UDC==1]
    (default) -> Motion_Mode.Start_Mode
    Motion_Mode.Normal_Mode -> Motion_Mode.Start_Mode : [speed<30]
  state Brake_Mode_Throttle
    entry: Engine_out=1;
    Motor_out=0;
    state Start_Mode
      entry: Brake_out=1;
    state Normal_Mode
      entry:Brake_out=0;
    (default) -> Brake_Mode_Throttle.Start_Mode
    Brake_Mode_Throttle.Start_Mode -> Brake_Mode_Throttle.Normal_Mode : [speed>=30&&UDC==1]
    Brake_Mode_Throttle.Normal_Mode -> Brake_Mode_Throttle.Start_Mode : [speed<30]
  (default) -> Motion_Mode
  Motion_Mode -> Brake_Mode_Throttle : [Brake_Pedal>0.05]
  Brake_Mode_Throttle -> Motion_Mode : [Brake_Pedal<0.05]
  data: speed input; acc input; Brake_Pedal input; Engine_out output; Motor_out output; UDC input; Brake_out output

== stateflow chart BTP_HEV_UDC_fInal_25_11_19/complete powertrain/Chart ==
  state GearShift
    state First
      Gear_number=1;
    state Second
      Gear_number=2;
    state Fifth
      Gear_number=5;
    state Third
      Gear_number=3;
    state Fourth
      Gear_number=4;
    (default) -> First
    First -> Second : [Vcl_Speed>13]
    Second -> First [order 1] : [Vcl_Speed<=13]
    Second -> Third [order 2] : [Vcl_Speed>20]
    Third -> Second [order 2] : [Vcl_Speed<=20]
    Fifth -> Fourth : [Vcl_Speed<=39]
    Fourth -> Fifth [order 2] : [Vcl_Speed>39]
    Third -> Fourth [order 1] : [Vcl_Speed>29]
    Fourth -> Third [order 1] : [Vcl_Speed<=29]
  (default) -> GearShift
  data: Vcl_Speed input; Gear_number output
